simulink model "S_example3"  (Simulink 7.5)
settings: Solver=ode4  StartTime=0.0  StopTime=10  FixedStep=0.001  RelTol=1e-3
values from neighbouring files (symbols this model uses):
  g = 9.8    [Intercept_cruise_fcn.m]    (also in S_example_3.m; result1.mat; result2.mat; result3.mat)
  L = 10.0    (= 10)    [S_example_3.m]    (also in result1.mat = 0.2; result2.mat = 0.5; result3.mat = 1; result4.mat = 5)
  m = 100    [Intercept_cruise_fcn.m]    (also in S_example_3.m = 1; result1.mat = 1; result2.mat = 1; result3.mat = 1)
settings Model: Creator=CT  LastModifiedBy=CT
settings DataIOCC: LimitDataPoints=off

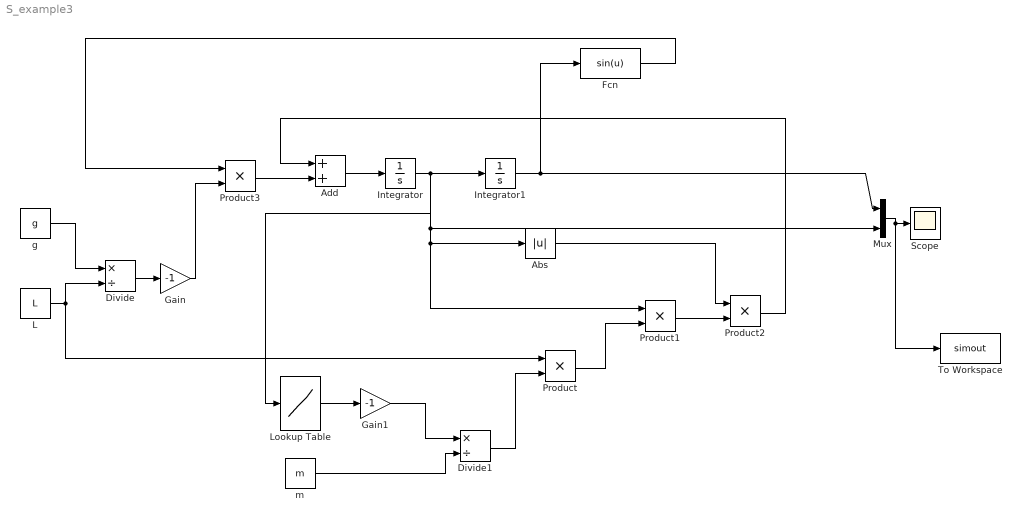
== system S_example3 ==
  Abs : Abs  OutDataType=fixdt(1, 16)  OutScaling=2^0
  Add : Sum  OutDataType=fixdt(1, 16)  OutScaling=2^-10
  Divide : Product  Inputs=*/  OutDataType=fixdt(1, 16)  OutScaling=2^-10
  Divide1 : Product  Inputs=*/  OutDataType=fixdt(1, 16)  OutScaling=2^-10
  Fcn : Fcn  Expr=sin(u)
  Gain : Gain  Gain=-1  ParameterDataType=fixdt(1, 16)  ParameterScaling=2^0  OutDataType=fixdt(1, 16)  OutScaling=2^0
  Gain1 : Gain  Gain=-1  ParameterDataType=fixdt(1, 16)  ParameterScaling=2^0  OutDataType=fixdt(1, 16)  OutScaling=2^0
  Integrator : Integrator
  Integrator1 : Integrator  InitialCondition=0.01
  L : Constant  Value=L  OutDataType=fixdt(1, 16)  OutScaling=2^0
  Lookup Table : Lookup  InputValues=[0.001 0.005 0.008 0.01 0.02]  Table=[0.1 0.11 0.14 0.2 0.5]  LookUpMeth=Interpolation-Use End Values  OutDataType=fixdt(1, 16)  OutScaling=2^0
  Mux : Mux  Inputs=2
  Product{,1..3} (4 alike) : Product  OutDataType=fixdt(1, 16)  OutScaling=2^0  RndMeth=Zero
  Scope : Scope
  To Workspace : ToWorkspace  VariableName=simout  SampleTime=-1  SaveFormat=Array
  g : Constant  Value=g  OutDataType=fixdt(1, 16)  OutScaling=2^0
  m : Constant  Value=m  OutDataType=fixdt(1, 16)  OutScaling=2^0
  wires:
  Integrator/1 -> Integrator1/1, Product1/1, Abs/1, Lookup Table/1, Mux/2
  g/1 -> Divide/1
  L/1 -> Divide/2, Product/1
  Lookup Table/1 -> Gain1/1
  m/1 -> Divide1/2
  Divide1/1 -> Product/2
  Product/1 -> Product1/2
  Product1/1 -> Product2/2
  Abs/1 -> Product2/1
  Product2/1 -> Add/1
  Mux/1 -> Scope/1, To Workspace/1
  Integrator1/1 -> Mux/1, Fcn/1
  Fcn/1 -> Product3/1
  Divide/1 -> Gain/1
  Gain/1 -> Product3/2
  Product3/1 -> Add/2
  Add/1 -> Integrator/1
  Gain1/1 -> Divide1/1
